simulink model "DTC_SV_R2013a"  (R2013a)
settings: Solver=ode3  StartTime=0.0  StopTime=1.1  FixedStep=Ts  MaxStep=20e-7  RelTol=1e-3
InitFcn:
  | Ts=10e-7;
  | psisx=0.996;
  | Vdc=600;
  | Ts_SVPWM=1e-4;
StopFcn:
  | plot(fs(:,1),fs(:,2),'-r',fr(:,1),fr(:,2),'-b');
  | axis equal;
  | grid on;
  | title('Flux Space Vector Trajectory');
  | text(.8,-.85,'rotor flux','color','b');
  | text(-1,-.85,'stator flux','color','r');
libraries: powerlib x12, powerlib_meascontrol x3, simulink_extras x3, simulink x2
Description:
  | Direct Torque Control (DTC) of Induction Motor (IM) Using Space Vector Pulse Width Modulation (SVPWM)
  | 
  | Pradipta Kumar Pal
  | Research Scholar,
  | Department of Electrical Engineering,
  | Indian Institute of Technology (Indian School of Mines), Dhanbad
settings Model: SimulationMode=accelerator  Creator=Pradipta Kumar Pal  LastModifiedBy=Pradipta
settings DataIOCC: SignalLoggingSaveFormat=ModelDataLogs  SignalLoggingName=sigsOut
settings OptimizationCC: BlockReduction=off  BooleanDataType=off  ExpressionDepthLimit=2147483647
settings DebuggingCC: SaveWithParameterizedLinksMsg=none  SignalResolutionControl=TryResolveAllWithWarning  SolverPrmCheckMsg=none  MultiTaskDSMMsg=warning  MultiTaskCondExecSysMsg=none  FcnCallInpInsideContextMsg=EnableAllAsWarning  FrameProcessingCompatibilityMsg=error  StrictBusMsg=ErrorOnBusTreatedAsVector
settings HardwareCC: TargetUnknown=on
settings GRTTargetCC: CodeReplacementLibrary=C89/C90 (ANSI)  CombineOutputUpdateFcns=off  GRTInterface=on
settings SimscapeCC: SimscapeNormalizeSystem=off
settings ConfigurationSet: Description=Simscape Multibody

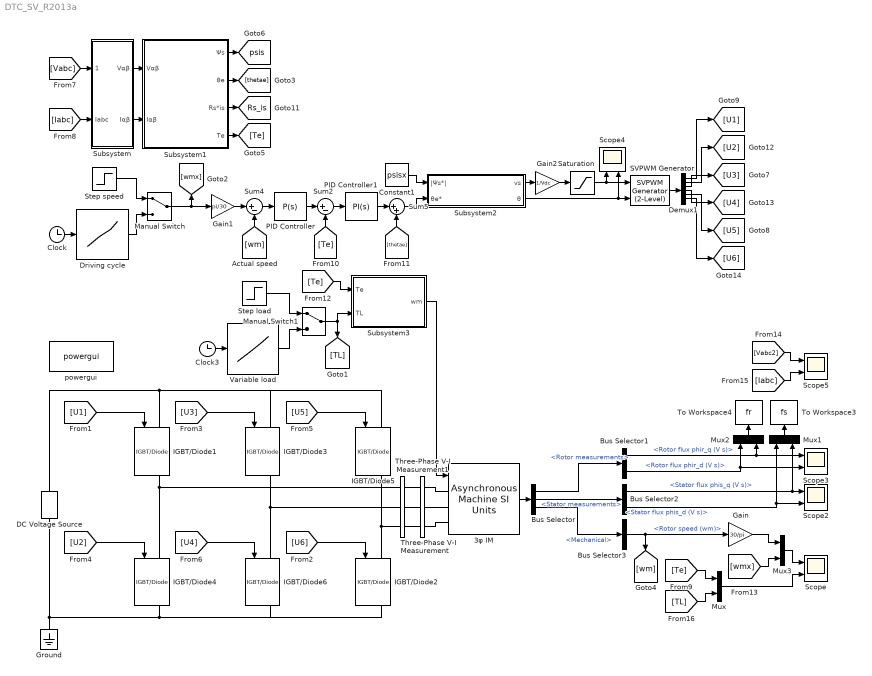
== system DTC_SV_R2013a ==
  3φ IM : powerlib/Machines/Asynchronous Machine SI Units  RotorType=Squirrel-cage  PresetModel="15:  5.4 HP (4KW)   400 V  50Hz 1430 RPM"  MechanicalLoad=Speed w  ShowDetailedParameters=on  ReferenceFrame=Stationary  Units=SI  MeasurementBus=off  NominalParameters=[4000 400 50]  Stator=[1.405 0.005839]  Rotor=[1.395 0.005839]  Cage1=[0.4155 0.002066]  Cage2=[0.4168 0.0003495]  Lm=0.1722  Mechanical=[0.0131 0.002985 2]  PolePairs=2  InitialConditions=[1 0 0 0 0 0 0 0]  SimulateSaturation=off  Saturation=[14.03593122, 27.81365428, 53.79336849, 72.68890987, 97.98006896, 148.6815601, 215.7428561, 302.9841135, 428.7778367 ; 230, 322, 414, 460, 506, 552, 598, 644, 690]  LoadFlowParameters=1492000  TsPowergui=0  TsBlock=-1  IterativeModel=Trapezoidal non iterative  IterativeDiscreteModel=Trapezoidal non iterative  Pmec=1.492e+006
  Bus Selector : BusSelector  OutputSignals=Rotor measurements,Stator measurements,Mechanical
  Bus Selector1 : BusSelector  OutputSignals=Rotor flux phir_q (V s),Rotor flux phir_d (V s)
  Bus Selector2 : BusSelector  OutputSignals=Stator flux phis_q (V s),Stator flux phis_d (V s)
  Bus Selector3 : BusSelector  OutputSignals=Rotor speed (wm)
  Clock : Clock
  Clock3 : Clock
  Constant1 : Constant  Value=psisx
  DC Voltage Source : powerlib/Electrical Sources/DC Voltage Source  Amplitude=Vdc  Measurements=None
  Demux1 : Demux  Outputs=6
  Driving cycle : Lookup_n-D  NumberOfTableDimensions=1  BreakpointsForDimension1=[0 1 2 5 5.001 8 8.001 10 11 12]/2  Table=[0 0 480 480 1430 1430 0 0 480 480]  RndMeth=Simplest  InputSameDT=on
  Gain : Gain  Gain=30/pi
  Gain1 : Gain  Gain=pi/30
  Gain2 : Gain  Gain=1/Vdc
  Ground : powerlib/Elements/Ground  LConnTagsString=a
  IGBT/Diode{1..6} (6 alike) : powerlib/Power Electronics/IGBT//Diode  Ron=1e-3  Rs=1e5  Cs=inf  Measurements=on
  Manual Switch : ManualSwitch
  Manual Switch1 : ManualSwitch
  Mux{,1..3} (4 alike) : Mux  Inputs=2
  PID Controller : simulink/Continuous/PID Controller  Controller=P  TimeDomain=Continuous-time  SampleTime=-1  IntegratorMethod=Forward Euler  FilterMethod=Forward Euler  Form=Parallel  UseFilter=on  ControllerParametersSource=internal  P=20  I=20  D=0  N=100  InitialConditionSource=internal  InitialConditionForIntegrator=0  InitialConditionForFilter=0  ExternalReset=none  LimitOutput=on  UpperSaturationLimit=30  LowerSaturationLimit=-30  LinearizeAsGain=on  AntiWindupMode=clamping  Kb=1  TrackingMode=off  Kt=1  PParamMin=[]  PParamMax=[]  IParamMin=[]  IParamMax=[]  DParamMin=[]  DParamMax=[]  NParamMin=[]  NParamMax=[]  KbParamMin=[]  KbParamMax=[]  KtParamMin=[]  KtParamMax=[]  POutMin=[]  POutMax=[]  IOutMin=[]  IOutMax=[]  DOutMin=[]  DOutMax=[]  NOutMin=[]  NOutMax=[]  KbOutMin=[]  KbOutMax=[]  KtOutMin=[]  KtOutMax=[]  IntegratorOutMin=[]  IntegratorOutMax=[]  FilterOutMin=[]  FilterOutMax=[]  SumOutMin=[]  SumOutMax=[]  SumI1OutMin=[]  SumI1OutMax=[]  SumI2OutMin=[]  SumI2OutMax=[]  SumI3OutMin=[]  SumI3OutMax=[]  SumDOutMin=[]  SumDOutMax=[]  SaturationOutMin=[]  SaturationOutMax=[]  IntegratorContinuousStateAttributes=''  IntegratorStateMustResolveToSignalObject=off  IntegratorRTWStateStorageClass=Auto  FilterContinuousStateAttributes=''  FilterStateMustResolveToSignalObject=off  FilterRTWStateStorageClass=Auto  DifferentiatorICPrevScaledInput=0  DifferentiatorOutMin=[]  DifferentiatorOutMax=[]
  PID Controller1 : simulink/Continuous/PID Controller  Controller=PI  TimeDomain=Continuous-time  SampleTime=-1  IntegratorMethod=Forward Euler  FilterMethod=Forward Euler  Form=Parallel  UseFilter=on  ControllerParametersSource=internal  P=0.005  I=1  D=0.00005  N=100  InitialConditionSource=internal  InitialConditionForIntegrator=0  InitialConditionForFilter=0  ExternalReset=none  LimitOutput=on  UpperSaturationLimit=pi/2  LowerSaturationLimit=-pi/2  LinearizeAsGain=on  AntiWindupMode=clamping  Kb=1  TrackingMode=off  Kt=1  PParamMin=[]  PParamMax=[]  IParamMin=[]  IParamMax=[]  DParamMin=[]  DParamMax=[]  NParamMin=[]  NParamMax=[]  KbParamMin=[]  KbParamMax=[]  KtParamMin=[]  KtParamMax=[]  POutMin=[]  POutMax=[]  IOutMin=[]  IOutMax=[]  DOutMin=[]  DOutMax=[]  NOutMin=[]  NOutMax=[]  KbOutMin=[]  KbOutMax=[]  KtOutMin=[]  KtOutMax=[]  IntegratorOutMin=[]  IntegratorOutMax=[]  FilterOutMin=[]  FilterOutMax=[]  SumOutMin=[]  SumOutMax=[]  SumI1OutMin=[]  SumI1OutMax=[]  SumI2OutMin=[]  SumI2OutMax=[]  SumI3OutMin=[]  SumI3OutMax=[]  SumDOutMin=[]  SumDOutMax=[]  SaturationOutMin=[]  SaturationOutMax=[]  IntegratorContinuousStateAttributes=''  IntegratorStateMustResolveToSignalObject=off  IntegratorRTWStateStorageClass=Auto  FilterContinuousStateAttributes=''  FilterStateMustResolveToSignalObject=off  FilterRTWStateStorageClass=Auto  DifferentiatorICPrevScaledInput=0  DifferentiatorOutMin=[]  DifferentiatorOutMax=[]
  SVPWM Generator : powerlib_meascontrol/Pulse & Signal Generators/SVPWM Generator (2-Level)  InputType=Magnitude-Angle (rad)  SwitchingPattern=Pattern #1  Fc=1/Ts_SVPWM  ParUref=[0.8 -30 50]  Ts=Ts
  Saturation : Saturate  UpperLimit=1  LowerLimit=0
  Scope{,2..5} (5 alike) : Scope  NumInputPorts=2
      Scope settings: TimeRange=auto  MaxDataPoints=5000  SaveToWorkspace=off  YMin=-150.00082~-3.93819  YMax=1350.00009~34.5966  SampleTime=-1
      Scope2 settings: TimeRange=auto  MaxDataPoints=5000  SaveToWorkspace=off  SaveName=ScopeData2  YMin=-1.24882~-1.24882  YMax=1.24881~1.24881  SampleTime=-1
      Scope3 settings: TimeRange=auto  MaxDataPoints=5000  SaveToWorkspace=off  SaveName=ScopeData3  YMin=-1.20226~-1.20226  YMax=1.20224~1.20224  SampleTime=-1
      Scope4 settings: TimeRange=auto  MaxDataPoints=5000  SaveToWorkspace=off  SaveName=ScopeData2  YMin=-0.12499~-3.92698  YMax=1.125~3.92699  SampleTime=-1
      Scope5 settings: TimeRange=auto  MaxDataPoints=5e4  SaveToWorkspace=off  YMin=-750.02667~-15.00000  YMax=750.02666~15.00000  SampleTime=-1
  Step load : Step  Time=0.9  After=12  SampleTime=0
  Step speed : Step  Time=0.15  After=1200  SampleTime=0
  Subsystem : Subsystem
      mask help: abc to αβ
      mask Display: disp('abc\nto\nαβ')
  Subsystem1 : Subsystem  mask{Rs=1.405}
      mask prompts: Rs "Stator resistance Rs (ohm)"
      mask help: Torque and Flux Estimator
      mask Display: disp('Flux and\nTorque\nEstimator')
  Subsystem2 : Subsystem  mask{Ts_SVPWM=Ts_SVPWM}
      mask prompts: Ts_SVPWM "SVPWM sampling time Ts (s)"
      mask help: dΨs/dt + Rs*is
      mask Display: disp('dΨs/dt + Rs*is')
  Subsystem3 : Subsystem  mask{J=0.0524, B=0.00597}
      mask prompts: J "Polar moment of inertia J (kg.m^2)"; B "Coefficient of viscous friction B (N.m.s)"
      mask help: Mechanical system
      mask Display: disp('Mechanical\nsystem')
  Sum2 : Sum  Inputs=|+-
  Sum4 : Sum  Inputs=|+-  SaturateOnIntegerOverflow=on  InputSameDT=on  OutDataTypeStr=Inherit: Same as first input
  Sum5 : Sum  Inputs=|++
  Three-Phase V-I Measurement : powerlib/Measurements/Three-Phase V-I Measurement  VoltageMeasurement=phase-to-ground  SetLabelV=on  LabelV=Vabc  Vpu=off  VpuLL=off  CurrentMeasurement=yes  SetLabelI=on  LabelI=Iabc  Ipu=off  Pbase=100e6  Vbase=500e3  OutputType=Complex  PhasorSimulation=off  PSBequivalent=0
  Three-Phase V-I Measurement1 : powerlib/Measurements/Three-Phase V-I Measurement  VoltageMeasurement=phase-to-phase  SetLabelV=on  LabelV=Vabc2  Vpu=off  VpuLL=off  CurrentMeasurement=no  SetLabelI=on  LabelI=Iabc  Ipu=off  Pbase=100e6  Vbase=500e3  OutputType=Complex  PhasorSimulation=off  PSBequivalent=0
  To Workspace3 : ToWorkspace  VariableName=fs  SampleTime=-1
      settings: Decimation=2
  To Workspace4 : ToWorkspace  VariableName=fr  SampleTime=-1
      settings: Decimation=2
  Variable load : Lookup_n-D  NumberOfTableDimensions=1  BreakpointsForDimension1=[0 3 4 12 13 14 17 18 20 21]/2  Table=[0 0 6 6 12 12 -6 -6 6 6]  RndMeth=Simplest  InputSameDT=on
  powergui : powerlib/powergui  Priority=1  SimulationMode=Discrete  SampleTime=Ts  frequency=60  Iterations=50  frequencyindice=50  Pbase=100e6  ErrMax=1e-4  UnitsV=kV  UnitsW=MW  buscounter=0  FunctionMessages=off  echomessages=off  EnableUseOfTLC=off  CurrentSourceSwitches=off  DisableSnubberDevices=off  DisableRonSwitches=off  DisableVfSwitches=off  DisplayEquations=off  SolverType=Tustin/Backward Euler (TBE)  Interpol=off  ExternalGateDelay=off  methode=off  Ts=100  x0status=blocks  SPID=off  SwTol=0  HookPort=off  RestoreLinks=warning  ResistiveCurrentMeasurement=off  Frange=[0:2:500]  Ylog=off  Xlog=on  ShowGrid=off  save=off  variable=ZData  structure=0  ZoomFFT=off  StartTime=0.0  cycles=1  DisplayStyle=1  fundamental=60  FreqAxis=off  MaxFrequency=1000  frequencyindicesteady=1  RmsSteady=1  display=off
  tag scope: Rs_is=global, psis=global
  wires:
  Sum4/1 -> PID Controller/1
  [U1] -> IGBT/Diode1/1
  [U3] -> IGBT/Diode3/1
  [U5] -> IGBT/Diode5/1
  [U2] -> IGBT/Diode4/1
  [U4] -> IGBT/Diode6/1
  [U6] -> IGBT/Diode2/1
  [Vabc2] -> Scope5/1
  [Iabc] -> Scope5/2
  Bus Selector/1 -> Bus Selector1/1  "<Rotor measurements>"
  Bus Selector3/1 -> Gain/1, [wm]  "<Rotor speed (wm)>"
  Bus Selector2/1 -> Scope2/1, Mux1/2  "<Stator flux phis_q (V s)>"
  [TL] -> Mux/2
  Mux3/1 -> Scope/1
  Bus Selector/3 -> Bus Selector3/1  "<Mechanical>"
  Mux1/1 -> To Workspace3/1
  Bus Selector1/2 -> Mux2/1, Scope3/2  "<Rotor flux phir_d (V s)>"
  [wmx] -> Mux3/2
  Mux/1 -> Scope/2
  Bus Selector2/2 -> Scope2/2, Mux1/1  "<Stator flux phis_d (V s)>"
  Mux2/1 -> To Workspace4/1
  Bus Selector1/1 -> Mux2/2, Scope3/1  "<Rotor flux phir_q (V s)>"
  Gain/1 -> Mux3/1
  3φ IM/1 -> Bus Selector/1
  Bus Selector/2 -> Bus Selector2/1  "<Stator measurements>"
  [Te] -> Mux/1
  [wm] -> Sum4/2
  Gain1/1 -> Sum4/1
  Demux1/1 -> [U1]
  Demux1/5 -> [U5]
  Demux1/3 -> [U3]
  Demux1/4 -> [U4]
  Demux1/2 -> [U2]
  SVPWM Generator/1 -> Demux1/1
  Demux1/6 -> [U6]
  Sum2/1 -> PID Controller1/1
  PID Controller/1 -> Sum2/1
  [Te] -> Sum2/2
  PID Controller1/1 -> Sum5/1
  [thetae] -> Sum5/2
  Manual Switch/1 -> [wmx], Gain1/1
  Clock/1 -> Driving cycle/1
  [Vabc] -> Subsystem/1(Vabc)
  [Iabc] -> Subsystem/2(Iabc)
  Subsystem/1(Vαβ) -> Subsystem1/1(Vαβ)
  Subsystem/2(Iαβ) -> Subsystem1/2(Iαβ)
  Subsystem1/1(Ψs) -> [psis]
  Subsystem1/2(θe) -> [thetae]
  Subsystem1/3(Rs*is) -> [Rs_is]
  Subsystem1/4(Te) -> [Te]
  Constant1/1 -> Subsystem2/1(|Ψs*|)
  Sum5/1 -> Subsystem2/2(θe*)
  Subsystem2/2(θ) -> Scope4/2, SVPWM Generator/2
  Gain2/1 -> Saturation/1
  Saturation/1 -> SVPWM Generator/1, Scope4/1
  Subsystem2/1(vs) -> Gain2/1
  Driving cycle/1 -> Manual Switch/2
  Step speed/1 -> Manual Switch/1
  Step load/1 -> Manual Switch1/1
  Variable load/1 -> Manual Switch1/2
  Clock3/1 -> Variable load/1
  Subsystem3/1(wm) -> 3φ IM/1
  Manual Switch1/1 -> [TL], Subsystem3/2(TL)
  [Te] -> Subsystem3/1(Te)
  connections:
  IGBT/Diode1/RConn1 -- Three-Phase V-I Measurement/LConn1 -- IGBT/Diode4/LConn1
  IGBT/Diode3/RConn1 -- Three-Phase V-I Measurement/LConn2 -- IGBT/Diode6/LConn1
  DC Voltage Source/RConn1 -- IGBT/Diode3/LConn1 -- IGBT/Diode5/LConn1 -- IGBT/Diode1/LConn1
  DC Voltage Source/LConn1 -- Ground/LConn1 -- IGBT/Diode2/RConn1 -- IGBT/Diode6/RConn1 -- IGBT/Diode4/RConn1
  IGBT/Diode2/LConn1 -- Three-Phase V-I Measurement/LConn3 -- IGBT/Diode5/RConn1
  3φ IM/LConn3 -- Three-Phase V-I Measurement1/RConn3
  Three-Phase V-I Measurement1/RConn2 -- 3φ IM/LConn2
  3φ IM/LConn1 -- Three-Phase V-I Measurement1/RConn1
  Three-Phase V-I Measurement/RConn1 -- Three-Phase V-I Measurement1/LConn1
  Three-Phase V-I Measurement/RConn2 -- Three-Phase V-I Measurement1/LConn2
  Three-Phase V-I Measurement/RConn3 -- Three-Phase V-I Measurement1/LConn3

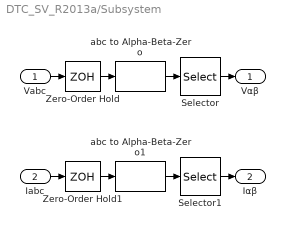
== system DTC_SV_R2013a/Subsystem ==
  Vabc : Inport
  Iabc : Inport  Port=2
  Selector : Selector  InputPortWidth=3  IndexOptions=Index vector (dialog)  Indices=[1 2]  OutputSizes=1
  Selector1 : Selector  InputPortWidth=3  IndexOptions=Index vector (dialog)  Indices=[1 2]  OutputSizes=1
  Zero-Order Hold : ZeroOrderHold  SampleTime=Ts
  Zero-Order Hold1 : ZeroOrderHold  SampleTime=Ts
  abc to Alpha-Beta-Zero : powerlib_meascontrol/Transformations/abc to Alpha-Beta-Zero
  abc to Alpha-Beta-Zero1 : powerlib_meascontrol/Transformations/abc to Alpha-Beta-Zero
  Vαβ : Outport
  Iαβ : Outport  Port=2
  wires:
  abc to Alpha-Beta-Zero/1 -> Selector/1
  Selector1/1 -> Iαβ/1
  Zero-Order Hold/1 -> abc to Alpha-Beta-Zero/1
  Vabc/1 -> Zero-Order Hold/1
  Selector/1 -> Vαβ/1
  Iabc/1 -> Zero-Order Hold1/1
  Zero-Order Hold1/1 -> abc to Alpha-Beta-Zero1/1
  abc to Alpha-Beta-Zero1/1 -> Selector1/1

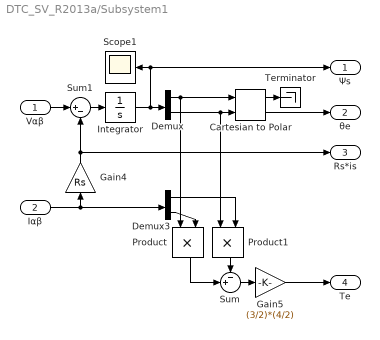
== system DTC_SV_R2013a/Subsystem1 ==
  Vαβ : Inport
  Iαβ : Inport  Port=2
  Cartesian to Polar : simulink_extras/Transformations/Cartesian to Polar
  Demux : Demux  Outputs=2
  Demux3 : Demux  Outputs=2
  Gain4 : Gain  Gain=Rs
  Gain5 : Gain  Gain=(3/2)*(4/2)
  Integrator : Integrator
  Product : Product
  Product1 : Product
  Scope1 : Scope
      settings: TimeRange=auto  MaxDataPoints=5000  SaveToWorkspace=off  YMin=-1.24748  YMax=1.24822  SampleTime=-1
  Sum : Sum  Inputs=-+|
  Sum1 : Sum  Inputs=|+-
  Terminator : Terminator
  Ψs : Outport
  θe : Outport  Port=2
  Rs*is : Outport  Port=3
  Te : Outport  Port=4
  wires:
  Vαβ/1 -> Sum1/1
  Integrator/1 -> Demux/1, Ψs/1, Scope1/1
  Sum1/1 -> Integrator/1
  Gain4/1 -> Rs*is/1, Sum1/2
  Demux3/1 -> Product1/2
  Demux3/2 -> Product/2
  Demux/2 -> Product1/1, Cartesian to Polar/2
  Product/1 -> Sum/2
  Cartesian to Polar/1 -> Terminator/1
  Demux/1 -> Cartesian to Polar/1, Product/1
  Sum/1 -> Gain5/1
  Product1/1 -> Sum/1
  Iαβ/1 -> Demux3/1, Gain4/1
  Gain5/1 -> Te/1
  Cartesian to Polar/2 -> θe/1

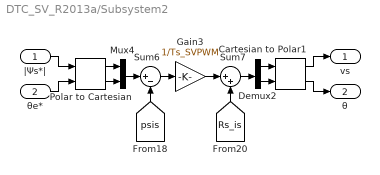
== system DTC_SV_R2013a/Subsystem2 ==
  |Ψs*| : Inport
  θe* : Inport  Port=2
  Cartesian to Polar1 : simulink_extras/Transformations/Cartesian to Polar
  Demux2 : Demux  Outputs=2
  Gain3 : Gain  Gain=1/Ts_SVPWM
  Mux4 : Mux  Inputs=2
  Polar to Cartesian : simulink_extras/Transformations/Polar to Cartesian
  Sum6 : Sum  Inputs=|+-
  Sum7 : Sum  Inputs=|++
  vs : Outport
  θ : Outport  Port=2
  wires:
  Mux4/1 -> Sum6/1
  |Ψs*|/1 -> Polar to Cartesian/1
  Gain3/1 -> Sum7/1
  Polar to Cartesian/2 -> Mux4/2
  Demux2/1 -> Cartesian to Polar1/1
  Sum6/1 -> Gain3/1
  Demux2/2 -> Cartesian to Polar1/2
  [psis] -> Sum6/2
  Polar to Cartesian/1 -> Mux4/1
  Sum7/1 -> Demux2/1
  [Rs_is] -> Sum7/2
  θe*/1 -> Polar to Cartesian/2
  Cartesian to Polar1/1 -> vs/1
  Cartesian to Polar1/2 -> θ/1

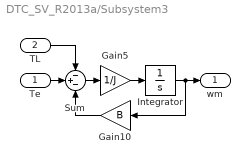
== system DTC_SV_R2013a/Subsystem3 ==
  Te : Inport
  TL : Inport  Port=2
  Gain10 : Gain  Gain=B
  Gain5 : Gain  Gain=1/J
  Integrator : Integrator
  Sum : Sum  Inputs=-+-
  wm : Outport
  wires:
  Sum/1 -> Gain5/1
  Te/1 -> Sum/2
  TL/1 -> Sum/1
  Gain5/1 -> Integrator/1
  Integrator/1 -> wm/1, Gain10/1
  Gain10/1 -> Sum/3
